simulink library "rot"  (R2024a)
settings: Solver=VariableStepAuto  StartTime=0.0  StopTime=10.0  RelTol=1e-3
undefined symbols (not defined in the file or in its folder): KFOC_PolePairs_p, KROT_SpdCutoffFreq_C
libraries: LibraryGRC x1
settings Model: Creator=FVT22063  LastModifiedBy=FVT22063
settings SFSimCC: SimCustomHeaderCode="#include \"FVTMC_API.h\""  SimUserSources=FVTMC_API.c

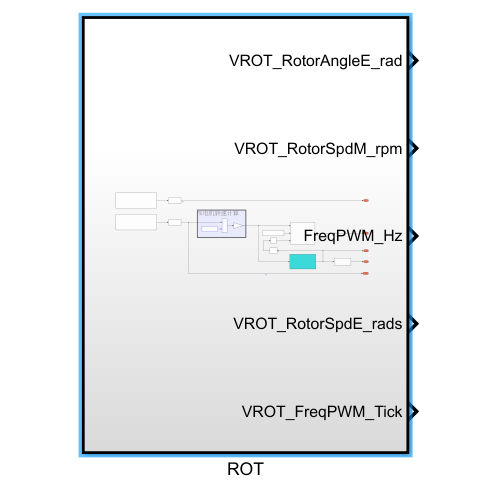
[thumbnail: Simulink's stored preview of the top-level diagram]
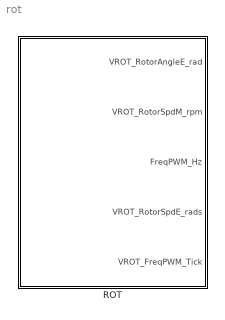
== system rot ==
  ROT : Subsystem  TreatAsAtomicUnit=on
      settings: RTWSystemCode=Nonreusable function  RTWFcnNameOpts=Use subsystem name  RTWFileNameOpts=Use subsystem name

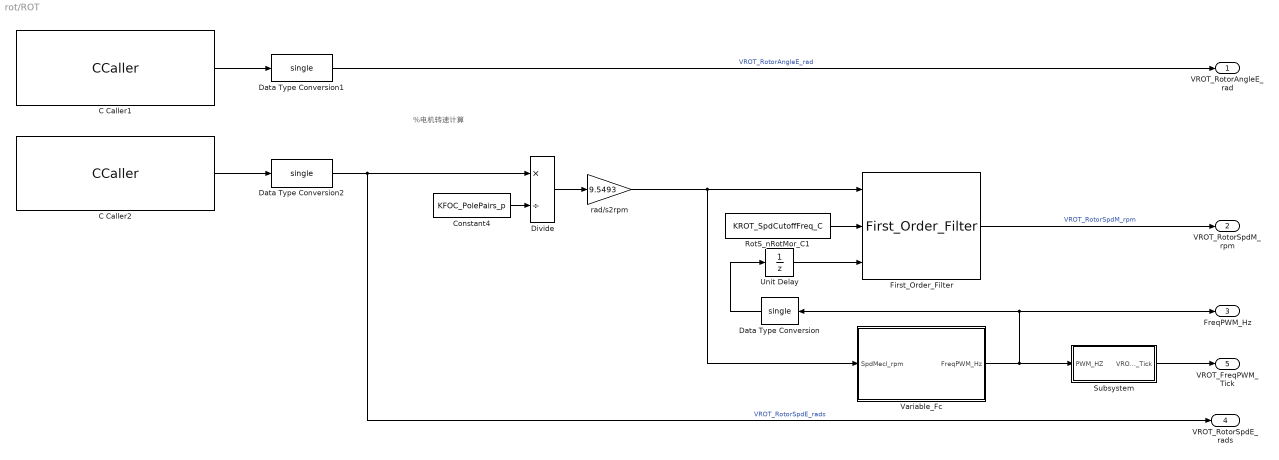
== system rot/ROT ==
  note: %电机转速计算
  C Caller1 : CCaller  FunctionName=rdc_get_lastest_electricalAngle  PortSpecificationStruct="%)30     .    & (   8    (     @         %    \"     $    !     0         %  0 \"0    $    _    07)G3F%M90  4&]R=$YA;64 4V-O<&4     26YD97@     5'EP90      4VEZ90      27-';&]B86P   X    P    !@    @    $          4    (     0    ,    !         !   P!O=70 #@   #     &    \"     0         !0    @    !     P    $         $  # &]U=  .    .     8    (    !          %    \"     $    &     0         0    !@   $]U='!U=   #@   #@    &    \"     8         !0    @    !     0    $         \"0    @               X    X    !@    @    $          4    (     0    8    !         !     &    <VEN9VQE   .    ,     8    (    !          %    \"     $    !     0         0  $ ,0    X    P    !@    @    ) @        4    (     0    $    !          (  0"
  C Caller2 : CCaller  FunctionName=rdc_get_lastest_speedRad  PortSpecificationStruct="%)30     .    & (   8    (     @         %    \"     $    !     0         %  0 \"0    $    _    07)G3F%M90  4&]R=$YA;64 4V-O<&4     26YD97@     5'EP90      4VEZ90      27-';&]B86P   X    P    !@    @    $          4    (     0    ,    !         !   P!O=70 #@   #     &    \"     0         !0    @    !     P    $         $  # &]U=  .    .     8    (    !          %    \"     $    &     0         0    !@   $]U='!U=   #@   #@    &    \"     8         !0    @    !     0    $         \"0    @               X    X    !@    @    $          4    (     0    8    !         !     &    <VEN9VQE   .    ,     8    (    !          %    \"     $    !     0         0  $ ,0    X    P    !@    @    ) @        4    (     0    $    !          (  0"
  Constant4 : Constant  Value=KFOC_PolePairs_p
  Data Type Conversion : DataTypeConversion  OutDataTypeStr=single  SaturateOnIntegerOverflow=off  RndMeth=Floor
  Data Type Conversion1 : DataTypeConversion  OutDataTypeStr=single  SaturateOnIntegerOverflow=off  RndMeth=Floor
  Data Type Conversion2 : DataTypeConversion  OutDataTypeStr=single  SaturateOnIntegerOverflow=off  RndMeth=Floor
  Divide : Product  Inputs=*/
  First_Order_Filter : LibraryGRC/First_Order_Filter  SystemSampleTime=-1  VariantActivationTime=update diagram  AllowFlexibleInterface=on  Latency=0  AutoFrameSizeCalculation=off
  RotS_nRotMor_C1 : Constant  Value=KROT_SpdCutoffFreq_C  OutDataTypeStr=single
  Subsystem : Subsystem
  Unit Delay : UnitDelay  InitialCondition=5000  SampleTime=-1  HasFrameUpgradeWarning=on
  Variable_Fc : Subsystem
  rad/s2rpm : Gain  Gain=9.5493
  VROT_RotorAngleE_rad : Outport  OutDataTypeStr=single  VectorParamsAs1DForOutWhenUnconnected=off
  VROT_RotorSpdM_rpm : Outport  Port=2  VectorParamsAs1DForOutWhenUnconnected=off
  FreqPWM_Hz : Outport  Port=3  VectorParamsAs1DForOutWhenUnconnected=off
  VROT_RotorSpdE_rads : Outport  Port=4  VectorParamsAs1DForOutWhenUnconnected=off
  VROT_FreqPWM_Tick : Outport  Port=5  VectorParamsAs1DForOutWhenUnconnected=off
  wires:
  C Caller2/1 -> Data Type Conversion2/1
  Unit Delay/1 -> First_Order_Filter/3
  rad/s2rpm/1 -> Variable_Fc/1(SpdMecl_rpm), First_Order_Filter/1
  First_Order_Filter/1 -> VROT_RotorSpdM_rpm/1  "VROT_RotorSpdM_rpm"
  RotS_nRotMor_C1/1 -> First_Order_Filter/2
  Variable_Fc/1(FreqPWM_Hz) -> Subsystem/1(PWM_HZ), FreqPWM_Hz/1, Data Type Conversion/1
  Divide/1 -> rad/s2rpm/1
  Data Type Conversion/1 -> Unit Delay/1
  Constant4/1 -> Divide/2
  C Caller1/1 -> Data Type Conversion1/1
  Data Type Conversion1/1 -> VROT_RotorAngleE_rad/1  "VROT_RotorAngleE_rad"
  Data Type Conversion2/1 -> Divide/1, VROT_RotorSpdE_rads/1  "VROT_RotorSpdE_rads"
  Subsystem/1(VROT_FreqPWM_Tick) -> VROT_FreqPWM_Tick/1

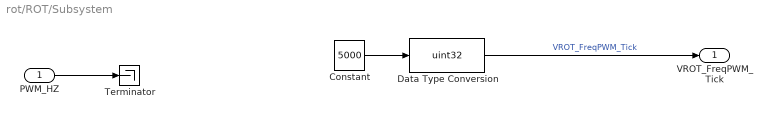
== system rot/ROT/Subsystem ==
  PWM_HZ : Inport
  Constant : Constant  Value=5000
  Data Type Conversion : DataTypeConversion  OutDataTypeStr=uint32  SaturateOnIntegerOverflow=off  RndMeth=Floor
  Terminator : Terminator
  VROT_FreqPWM_Tick : Outport
  wires:
  Constant/1 -> Data Type Conversion/1
  Data Type Conversion/1 -> VROT_FreqPWM_Tick/1  "VROT_FreqPWM_Tick"
  PWM_HZ/1 -> Terminator/1

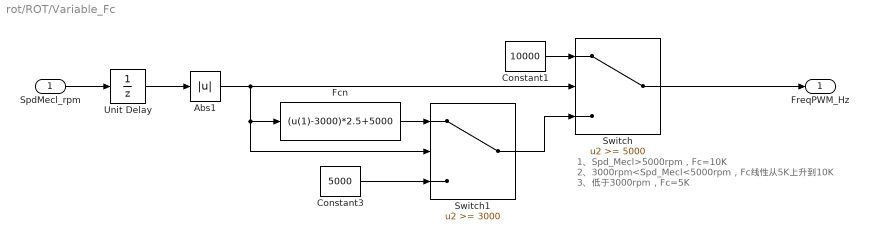
== system rot/ROT/Variable_Fc ==
  note: 1、Spd_Mecl>5000rpm，Fc=10K
      | 2、3000rpm<Spd_Mecl<5000rpm，Fc线性从5K上升到10K
      | 3、低于3000rpm，Fc=5K
  SpdMecl_rpm : Inport  OutDataTypeStr=single
  Abs1 : Abs  SaturateOnIntegerOverflow=off
  Constant1 : Constant  Value=10000  OutDataTypeStr=single
  Constant3 : Constant  Value=5000  OutDataTypeStr=single
  Fcn : Fcn  Expr=(u(1)-3000)*2.5+5000
  Switch : Switch  Threshold=5000  SaturateOnIntegerOverflow=off  InputSameDT=off
  Switch1 : Switch  Threshold=3000  SaturateOnIntegerOverflow=off  InputSameDT=off
  Unit Delay : UnitDelay  SampleTime=-1  HasFrameUpgradeWarning=on
  FreqPWM_Hz : Outport  OutDataTypeStr=single  VectorParamsAs1DForOutWhenUnconnected=off
  wires:
  SpdMecl_rpm/1 -> Unit Delay/1
  Unit Delay/1 -> Abs1/1
  Abs1/1 -> Fcn/1, Switch1/2, Switch/2
  Constant1/1 -> Switch/1
  Switch1/1 -> Switch/3
  Fcn/1 -> Switch1/1
  Constant3/1 -> Switch1/3
  Switch/1 -> FreqPWM_Hz/1
